simulink model "relay_tech"  (R2015a)
settings: Solver=ode3  StartTime=0.0  StopTime=300  FixedStep=0.1  RelTol=1e-3
settings Model: Creator=Caroline  LastModifiedBy=Caroline

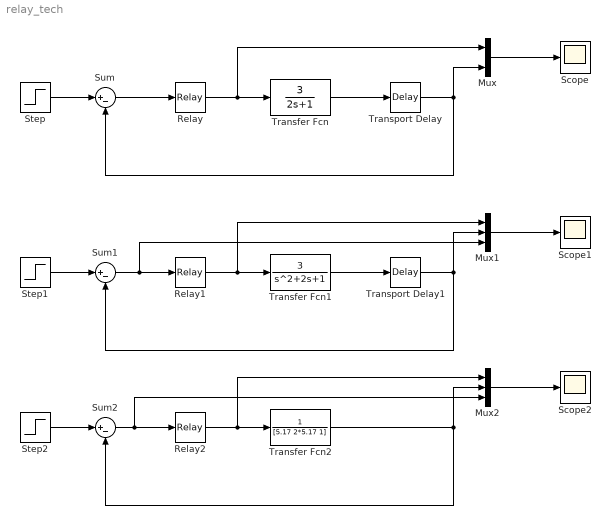
== system relay_tech ==
  Mux : Mux  Inputs=2
  Mux1 : Mux  Inputs=3
  Mux2 : Mux  Inputs=3
  Relay : Relay  OnSwitchValue=0.6  OffSwitchValue=-0.4  OnOutputValue=0.8  OffOutputValue=-0.2
  Relay1 : Relay  OnSwitchValue=0.5+0.15  OffSwitchValue=0.5-0.15  OffOutputValue=-1
  Relay2 : Relay  OnSwitchValue=0.3  OffSwitchValue=-0.3  OnOutputValue=2  OffOutputValue=-0.5
  Scope : Scope
      settings: ShowLegends=on
  Scope1 : Scope
      settings: ShowLegends=on  SaveName=ScopeData2
  Scope2 : Scope
      settings: ShowLegends=on  SaveName=ScopeData3
  Step : Step  SampleTime=0
  Step1 : Step  SampleTime=0
  Step2 : Step  SampleTime=0
  Sum : Sum  Inputs=|+-
  Sum1 : Sum  Inputs=|+-
  Sum2 : Sum  Inputs=|+-
  Transfer Fcn : TransferFcn  Numerator=[3]  Denominator=[2 1]
  Transfer Fcn1 : TransferFcn  Numerator=[3]
  Transfer Fcn2 : TransferFcn  Denominator=[5.17 2*5.17 1]
  Transport Delay : TransportDelay  DelayTime=0.1
  Transport Delay1 : TransportDelay  DelayTime=0.5
  wires:
  Step/1 -> Sum/1
  Sum/1 -> Relay/1
  Relay/1 -> Mux/1, Transfer Fcn/1
  Transfer Fcn/1 -> Transport Delay/1
  Transport Delay/1 -> Mux/2, Sum/2
  Mux/1 -> Scope/1
  Step1/1 -> Sum1/1
  Sum1/1 -> Mux1/3, Relay1/1
  Relay1/1 -> Mux1/1, Transfer Fcn1/1
  Transfer Fcn1/1 -> Transport Delay1/1
  Transport Delay1/1 -> Sum1/2, Mux1/2
  Mux1/1 -> Scope1/1
  Step2/1 -> Sum2/1
  Sum2/1 -> Mux2/3, Relay2/1
  Relay2/1 -> Mux2/1, Transfer Fcn2/1
  Transfer Fcn2/1 -> Sum2/2, Mux2/2
  Mux2/1 -> Scope2/1
